simulink model "HUAUV3_"  (R2019a)
settings: Solver=VariableStepAuto  StartTime=0.0  StopTime=30  RelTol=1e-3
InitFcn:
  | run('HUAUVInitial.m')
values from neighbouring files (symbols this model uses):
  buoPos =     [HUAUVPARAMETERS.mat]
  coeff =     [HUAUVPARAMETERS.mat]
  g = 9.8    [HUAUVInitial.m]    (also in HUAUVPARAMETERS.mat)
  Jx = 2.365e-2    (= 0.02365)    [HUAUVInitial.m]    (also in HUAUVPARAMETERS.mat)
  Jy = 1.318e-2    (= 0.01318)    [HUAUVInitial.m]    (also in HUAUVPARAMETERS.mat)
  Jz = 1.318e-2    (= 0.01318)    [HUAUVInitial.m]    (also in HUAUVPARAMETERS.mat)
  m = 1.8    [HUAUVInitial.m]    (also in HUAUVPARAMETERS.mat)
  Sx = 0.07*0.15    (= 0.0105)    [HUAUVInitial.m]    (also in HUAUVPARAMETERS.mat)
  Sy = 0.07*0.28    (= 0.0196)    [HUAUVInitial.m]    (also in HUAUVPARAMETERS.mat)
  Sz = 0.15*0.28    (= 0.042)    [HUAUVInitial.m]    (also in HUAUVPARAMETERS.mat)
  V = 1e-3    (= 0.001)    [HUAUVInitial.m]
undefined symbols (not defined in the file or in its folder): rho
libraries: simulink x12, shared6dof x2
(part 1 of 2)
settings Model: Creator=MI  LastModifiedBy=MI
settings DataIOCC: ReturnWorkspaceOutputs=off
settings DebuggingCC: PregeneratedLibrarySubsystemCodeDiagnostic=none  ArithmeticOperatorsInVariantConditions=warning
settings SFSimCC: SimUseLocalCustomCode=off
settings RTWCC: RTWUseLocalCustomCode=off

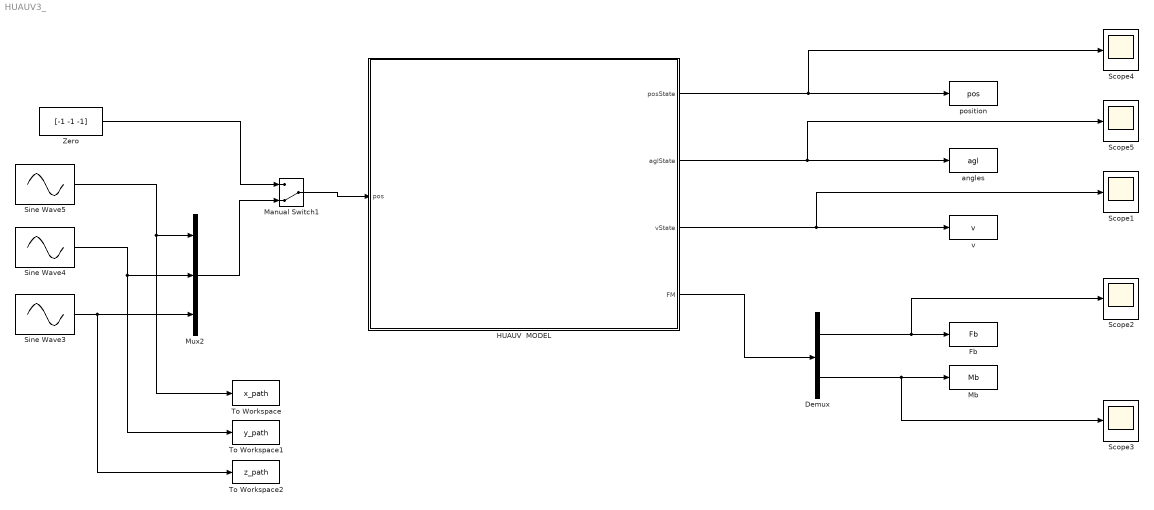
== system HUAUV3_ ==
  Demux : Demux  Outputs=2
  Fb : ToWorkspace  VariableName=Fb  SampleTime=-1
  HUAUV  MODEL : Subsystem
  Manual Switch1 : ManualSwitch  CurrentSetting=0
  Mb : ToWorkspace  VariableName=Mb  SampleTime=-1
  Mux2 : Mux  Inputs=3
  Scope{1..5} (5 alike) : Scope
  Sine Wave3 : Sin  Bias=1  Frequency=0.5  SampleTime=0
  Sine Wave4 : Sin  Frequency=2  Phase=pi/2  SampleTime=0
  Sine Wave5 : Sin  Frequency=2  Phase=pi/3  SampleTime=0
  To Workspace : ToWorkspace  VariableName=x_path  SampleTime=-1
  To Workspace1 : ToWorkspace  VariableName=y_path  SampleTime=-1
  To Workspace2 : ToWorkspace  VariableName=z_path  SampleTime=-1
  Zero : Constant  Value=[-1 -1 -1]
  angles : ToWorkspace  VariableName=agl  SampleTime=-1
  position : ToWorkspace  VariableName=pos  SampleTime=-1
  v : ToWorkspace  VariableName=v  SampleTime=-1
  wires:
  Manual Switch1/1 -> HUAUV  MODEL/1(pos)
  Sine Wave5/1 -> To Workspace/1, Mux2/1
  Sine Wave4/1 -> To Workspace1/1, Mux2/2
  Zero/1 -> Manual Switch1/1
  Mux2/1 -> Manual Switch1/2
  Sine Wave3/1 -> To Workspace2/1, Mux2/3
  HUAUV  MODEL/1(posState) -> position/1, Scope4/1
  HUAUV  MODEL/2(aglState) -> Scope5/1, angles/1
  HUAUV  MODEL/3(vState) -> Scope1/1, v/1
  HUAUV  MODEL/4(FM) -> Demux/1
  Demux/1 -> Scope2/1, Fb/1
  Demux/2 -> Scope3/1, Mb/1

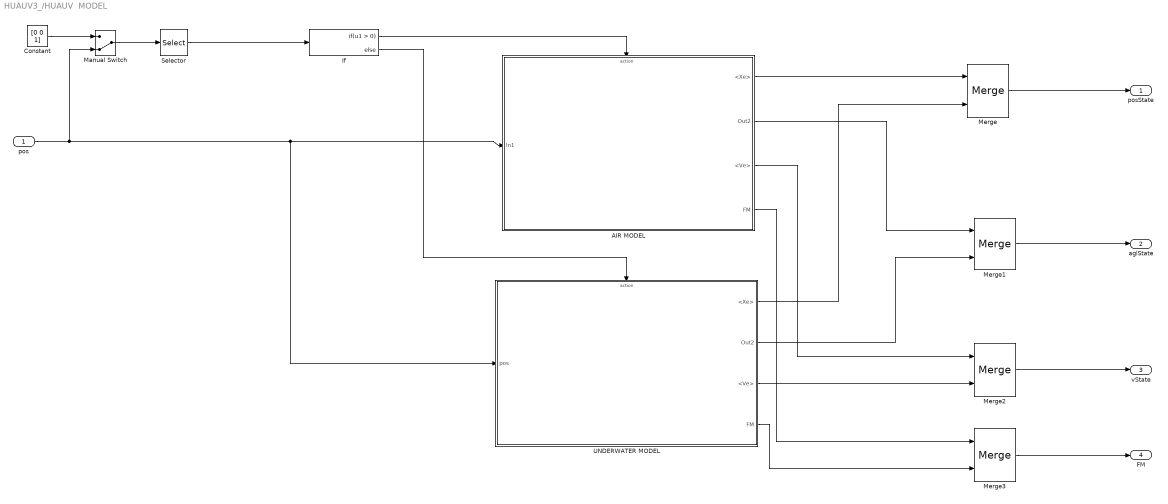
== system HUAUV3_/HUAUV  MODEL ==
  pos : Inport
  AIR MODEL : Subsystem
  Constant : Constant  Value=[0 0 1]
  If : If
  Manual Switch : ManualSwitch  CurrentSetting=0
  Merge{,1..3} (4 alike) : Merge
  Selector : Selector  InputPortWidth=3  IndexOptions=Index vector (dialog)  Indices=[3]  OutputSizes=1
  UNDERWATER MODEL : Subsystem
  posState : Outport
  aglState : Outport  Port=2
  vState : Outport  Port=3
  FM : Outport  Port=4
  wires:
  pos/1 -> Manual Switch/2, UNDERWATER MODEL/1(pos), AIR MODEL/1(In1)
  AIR MODEL/1(<Xe>) -> Merge/1
  UNDERWATER MODEL/1(<Xe>) -> Merge/2
  AIR MODEL/2(Out2) -> Merge1/1
  UNDERWATER MODEL/2(Out2) -> Merge1/2
  Merge1/1 -> aglState/1
  If/1 -> AIR MODEL/Action
  If/2 -> UNDERWATER MODEL/Action
  Manual Switch/1 -> Selector/1
  Merge/1 -> posState/1
  Selector/1 -> If/1
  Constant/1 -> Manual Switch/1
  AIR MODEL/3(<Ve>) -> Merge2/1
  UNDERWATER MODEL/3(<Ve>) -> Merge2/2
  Merge2/1 -> vState/1
  AIR MODEL/4(FM) -> Merge3/1
  UNDERWATER MODEL/4(FM) -> Merge3/2
  Merge3/1 -> FM/1

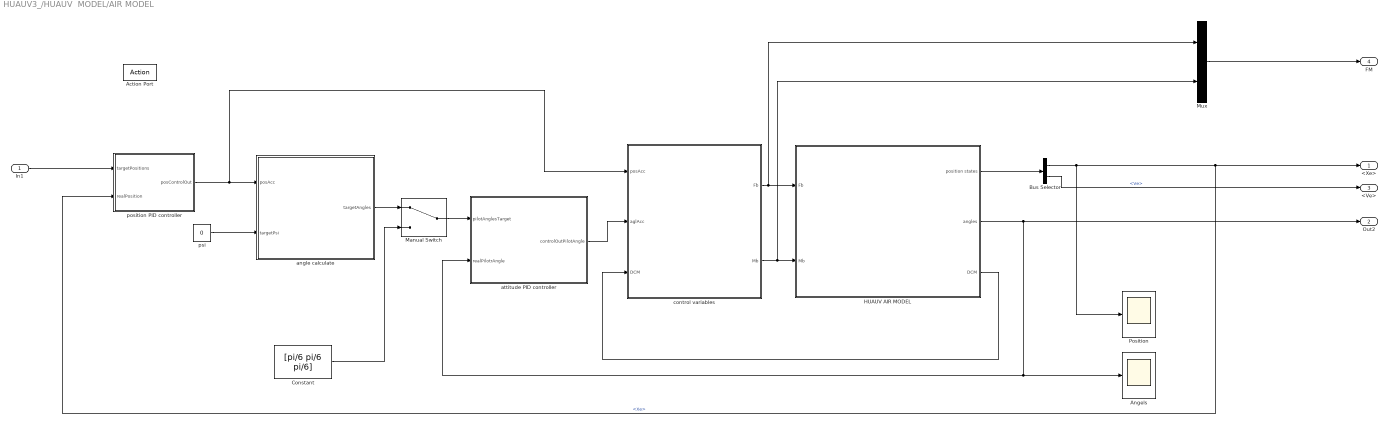
== system HUAUV3_/HUAUV  MODEL/AIR MODEL ==
  In1 : Inport
  Action Port : ActionPort  InitializeStates=reset  ActionPortLabel=if(u1 > 0)
  Angels : Scope
  Bus Selector : BusSelector  OutputSignals=Xe,Ve
  Constant : Constant  Value=[pi/6 pi/6 pi/6]
  HUAUV AIR MODEL : Subsystem
  Manual Switch : ManualSwitch
  Mux : Mux  Inputs=2
  Position : Scope
  angle calculate : Subsystem
  attitude PID controller : Subsystem
  control variables : Subsystem
  position PID controller : Subsystem
  psi : Constant  Value=0
  <Xe> : Outport
  Out2 : Outport  Port=2
  <Ve> : Outport  Port=3
  FM : Outport  Port=4
  wires:
  attitude PID controller/1(controlOutPilotAngle) -> control variables/2(aglAcc)
  position PID controller/1(posControlOut) -> control variables/1(posAcc), angle calculate/1(posAcc)
  psi/1 -> angle calculate/2(targetPsi)
  HUAUV AIR MODEL/1(position states) -> Bus Selector/1
  Constant/1 -> Manual Switch/2
  HUAUV AIR MODEL/3(DCM) -> control variables/3(DCM)
  control variables/2(Mb) -> Mux/2, HUAUV AIR MODEL/2(Mb)
  Manual Switch/1 -> attitude PID controller/1(pilotAnglesTarget)
  HUAUV AIR MODEL/2(angles) -> Out2/1, Angels/1, attitude PID controller/2(realPilotrAngle)
  Bus Selector/1 -> Position/1, position PID controller/2(realPosition), <Xe>/1  "<Xe>"
  angle calculate/1(targetAngles) -> Manual Switch/1
  In1/1 -> position PID controller/1(targetPositions)
  control variables/1(Fb) -> Mux/1, HUAUV AIR MODEL/1(Fb)
  Bus Selector/2 -> <Ve>/1  "<Ve>"
  Mux/1 -> FM/1

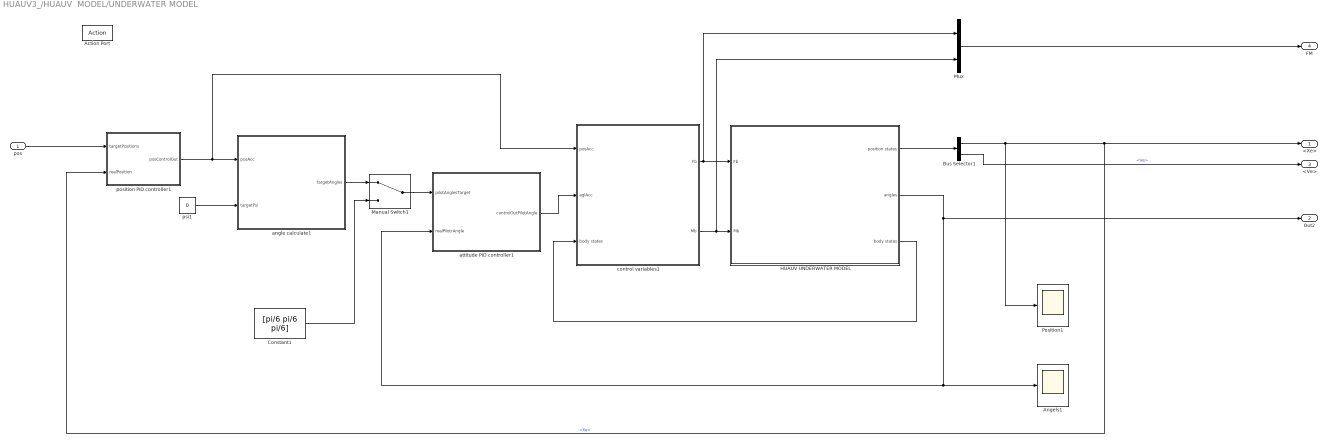
== system HUAUV3_/HUAUV  MODEL/UNDERWATER MODEL ==
  pos : Inport
  Action Port : ActionPort  InitializeStates=reset  ActionPortLabel=else
  Angels1 : Scope
  Bus Selector1 : BusSelector  OutputSignals=Xe,Ve
  Constant1 : Constant  Value=[pi/6 pi/6 pi/6]
  HUAUV UNDERWATER MODEL : Subsystem
  Manual Switch1 : ManualSwitch
  Mux : Mux  Inputs=2
  Position1 : Scope
  angle calculate1 : Subsystem
  attitude PID controller1 : Subsystem
  control variables1 : Subsystem
  position PID controller1 : Subsystem
  psi1 : Constant  Value=0
  <Xe> : Outport
  Out2 : Outport  Port=2
  <Ve> : Outport  Port=3
  FM : Outport  Port=4
  wires:
  position PID controller1/1(posControlOut) -> control variables1/1(posAcc), angle calculate1/1(posAcc)
  HUAUV UNDERWATER MODEL/2(angles) -> Out2/1, Angels1/1, attitude PID controller1/2(realPilotrAngle)
  HUAUV UNDERWATER MODEL/1(position states) -> Bus Selector1/1
  control variables1/1(Fb) -> Mux/1, HUAUV UNDERWATER MODEL/1(Fb)
  psi1/1 -> angle calculate1/2(targetPsi)
  angle calculate1/1(targetAngles) -> Manual Switch1/1
  control variables1/2(Mb) -> Mux/2, HUAUV UNDERWATER MODEL/2(Mb)
  HUAUV UNDERWATER MODEL/3(body states) -> control variables1/3(body states)
  Constant1/1 -> Manual Switch1/2
  attitude PID controller1/1(controlOutPilotAngle) -> control variables1/2(aglAcc)
  Bus Selector1/1 -> Position1/1, position PID controller1/2(realPosition), <Xe>/1  "<Xe>"
  Manual Switch1/1 -> attitude PID controller1/1(pilotAnglesTarget)
  pos/1 -> position PID controller1/1(targetPositions)
  Bus Selector1/2 -> <Ve>/1  "<Ve>"
  Mux/1 -> FM/1

== system HUAUV3_/HUAUV  MODEL/AIR MODEL/HUAUV AIR MODEL ==
  Fb : Inport
  Mb : Inport  Port=2
  Bus Creator : BusCreator  Inputs=3
  HUAUV  6DOF Dynamic Model (Euler Angles) : shared6dof/6DOF (Euler Angles)  units=Metric (MKS)  mtype=Custom Variable  rep=Euler Angles  xme_0=[0 0 0]  Vm_0=[0 0 0]  eul_0=[0 0 0]  pm_0=[0 0 0]  mass_0=1.0  mass_e=0.5  mass_f=2.0  inertia=eye(3)  inertia_e=eye(3)  inertia_f=2*eye(3)  k_quat=1.0  vre_flag=off  abi_flag=on  aMode=0  xme_statename=''  Vm_statename=''  eul_statename=''  quat_statename=''  pm_statename=''  mass_statename=''
      settings: SourceProductBaseCode=AE
  Terminator{1..4} (4 alike) : Terminator
  frame parameters : Subsystem
  position states : Outport
  angles : Outport  Port=2
  DCM : Outport  Port=3
  wires:
  HUAUV  6DOF Dynamic Model (Euler Angles)/2 -> Bus Creator/1  "Xe"
  HUAUV  6DOF Dynamic Model (Euler Angles)/4 -> DCM/1
  HUAUV  6DOF Dynamic Model (Euler Angles)/9 -> Bus Creator/3  "Ae"
  frame parameters/1(m) -> HUAUV  6DOF Dynamic Model (Euler Angles)/3
  HUAUV  6DOF Dynamic Model (Euler Angles)/1 -> Bus Creator/2  "Ve"
  HUAUV  6DOF Dynamic Model (Euler Angles)/7 -> Terminator3/1
  HUAUV  6DOF Dynamic Model (Euler Angles)/5 -> Terminator1/1
  HUAUV  6DOF Dynamic Model (Euler Angles)/8 -> Terminator4/1
  Mb/1 -> HUAUV  6DOF Dynamic Model (Euler Angles)/2
  Bus Creator/1 -> position states/1
  HUAUV  6DOF Dynamic Model (Euler Angles)/6 -> Terminator2/1
  frame parameters/2(dI/dt) -> HUAUV  6DOF Dynamic Model (Euler Angles)/4
  frame parameters/3(I) -> HUAUV  6DOF Dynamic Model (Euler Angles)/5
  Fb/1 -> HUAUV  6DOF Dynamic Model (Euler Angles)/1
  HUAUV  6DOF Dynamic Model (Euler Angles)/3 -> angles/1

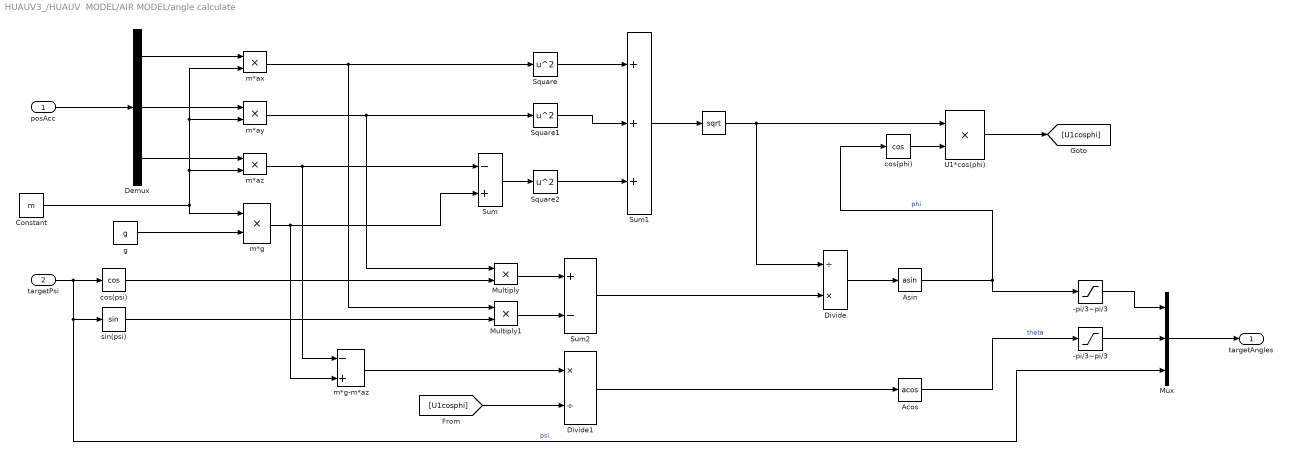
== system HUAUV3_/HUAUV  MODEL/AIR MODEL/angle calculate ==
  posAcc : Inport
  targetPsi : Inport  Port=2
  " " : Sqrt  SaturateOnIntegerOverflow=on
  -pi/3~pi/3 : Saturate  UpperLimit=pi/3  LowerLimit=-pi/3
  "-pi/3~pi/3  " : Saturate  UpperLimit=pi/3  LowerLimit=-pi/3
  Acos : Trigonometry  Operator=acos
  Asin : Trigonometry  Operator=asin
  Constant : Constant  Value=m
  Demux : Demux  Outputs=3
  Divide : Product  Inputs=/*
  Divide1 : Product  Inputs=*/
  Multiply : Product
  Multiply1 : Product
  Mux : Mux  Inputs=3
  Square : Math  Operator=square  SaturateOnIntegerOverflow=on
  Square1 : Math  Operator=square  SaturateOnIntegerOverflow=on
  Square2 : Math  Operator=square  SaturateOnIntegerOverflow=on
  Sum : Sum  Inputs=-+
  Sum1 : Sum  Inputs=+++
  Sum2 : Sum  Inputs=+-
  U1*cos(phi) : Product
  cos(phi) : Trigonometry  Operator=cos
  cos(psi) : Trigonometry  Operator=cos
  g : Constant  Value=g
  m*ax : Product
  m*ay : Product
  m*az : Product
  m*g : Product
  m*g-m*az : Sum  Inputs=-+
  sin(psi) : Trigonometry
  targetAngles : Outport
  wires:
  posAcc/1 -> Demux/1
  Demux/3 -> m*az/1
  Demux/2 -> m*ay/1
  Demux/1 -> m*ax/1
  Constant/1 -> m*g/1, m*ax/2, m*ay/2, m*az/2
  m*ay/1 -> Square1/1, Multiply/1
  m*ax/1 -> Multiply1/1, Square/1
  g/1 -> m*g/2
  m*g/1 -> m*g-m*az/2, Sum/2
  m*az/1 -> m*g-m*az/1, Sum/1
  Sum/1 -> Square2/1
  Square/1 -> Sum1/1
  Square2/1 -> Sum1/3
  Square1/1 -> Sum1/2
  Sum1/1 -> " "/1
  targetPsi/1 -> Mux/3, sin(psi)/1, cos(psi)/1  "psi"
  cos(psi)/1 -> Multiply/2
  sin(psi)/1 -> Multiply1/2
  Multiply1/1 -> Sum2/2
  Multiply/1 -> Sum2/1
  Sum2/1 -> Divide/2
  " "/1 -> Divide/1, U1*cos(phi)/1
  Divide/1 -> Asin/1
  Asin/1 -> -pi/3~pi/3/1, cos(phi)/1  "phi"
  Mux/1 -> targetAngles/1
  Acos/1 -> "-pi/3~pi/3  "/1  "theta"
  cos(phi)/1 -> U1*cos(phi)/2
  U1*cos(phi)/1 -> [U1cosphi]
  m*g-m*az/1 -> Divide1/1
  [U1cosphi] -> Divide1/2
  Divide1/1 -> Acos/1
  -pi/3~pi/3/1 -> Mux/1
  "-pi/3~pi/3  "/1 -> Mux/2

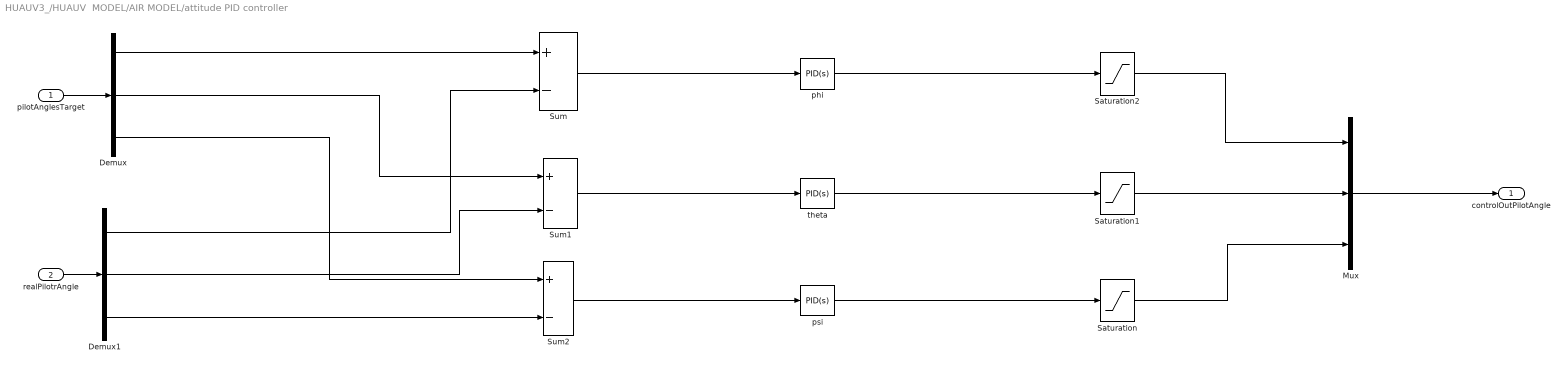
== system HUAUV3_/HUAUV  MODEL/AIR MODEL/attitude PID controller ==
  pilotAnglesTarget : Inport
  realPilotrAngle : Inport  Port=2
  Demux : Demux  Outputs=3
  Demux1 : Demux  Outputs=3
  Mux : Mux  Inputs=3
  Saturation : Saturate  UpperLimit=200  LowerLimit=-200
  Saturation1 : Saturate  UpperLimit=200  LowerLimit=-200
  Saturation2 : Saturate  UpperLimit=200  LowerLimit=-200
  Sum : Sum  Inputs=+-
  Sum1 : Sum  Inputs=+-
  Sum2 : Sum  Inputs=+-
  phi : simulink/Continuous/PID Controller  Controller=PID  Form=Parallel  TimeDomain=Continuous-time  SampleTime=-1  IntegratorMethod=Forward Euler  FilterMethod=Forward Euler  ControllerParametersSource=internal  P=607.007237650316  I=538.5363122748  D=152.017546187089  UseFilter=on  N=17379.6431323802  TunerSelectOption=Transfer Function Based (PID Tuner App)  InitialConditionSource=internal  InitialConditionForIntegrator=0  InitialConditionForFilter=0  DifferentiatorICPrevScaledInput=0  ExternalReset=none  TrackingMode=off  Kt=1  LimitOutput=off  UpperSaturationLimit=inf  LowerSaturationLimit=-inf  LinearizeAsGain=on  AntiWindupMode=none  Kb=1  POutMin=[]  POutMax=[]  IOutMin=[]  IOutMax=[]  DOutMin=[]  DOutMax=[]  NOutMin=[]  NOutMax=[]  SumOutMin=[]  SumOutMax=[]  SaturationOutMin=[]  SaturationOutMax=[]  PParamMin=[]  PParamMax=[]  IParamMin=[]  IParamMax=[]  DParamMin=[]  DParamMax=[]  NParamMin=[]  NParamMax=[]  KbParamMin=[]  KbParamMax=[]  KtParamMin=[]  KtParamMax=[]  KbOutMin=[]  KbOutMax=[]  KtOutMin=[]  KtOutMax=[]  IntegratorOutMin=[]  IntegratorOutMax=[]  FilterOutMin=[]  FilterOutMax=[]  SumI1OutMin=[]  SumI1OutMax=[]  SumI2OutMin=[]  SumI2OutMax=[]  SumI3OutMin=[]  SumI3OutMax=[]  SumI4OutMin=[]  SumI4OutMax=[]  SumDOutMin=[]  SumDOutMax=[]  DifferentiatorOutMin=[]  DifferentiatorOutMax=[]  FilterDiffOutCoefMin=[]  FilterDiffOutCoefMax=[]  ReciprocalOutMin=[]  ReciprocalOutMax=[]  SumDenOutMin=[]  SumDenOutMax=[]  SumNumOutMin=[]  SumNumOutMax=[]  DivideOutMin=[]  DivideOutMax=[]  IntegratorContinuousStateAttributes=''  IntegratorStateMustResolveToSignalObject=off  IntegratorRTWStateStorageClass=Auto  FilterContinuousStateAttributes=''  FilterStateMustResolveToSignalObject=off  FilterRTWStateStorageClass=Auto  ParallelPVariant=InternalParameters  IdealPVariant=Disabled  IVariant=InternalParameters  DVariant=InternalParameters  IntegratorVariant=Continuous  SatVariant=Disabled  AWVariant=Passthrough  PCopyVariant=Disabled  TRVariant=Disabled  FdbkBlocksVariant=Forward  IdealPFdbkVariant=Disabled  SatFdbkVariant=Disabled  DerivativeFilterVariant=ContFilter  NVariant=InternalParameters  NCopyVariant=Disabled  FilterICVariant=InternalICsFilter  IntegratorICVariant=InternalICs  ExternalResetVariant=Disabled  TRSumVariant=Passthrough  SumFdbkVariant=Disabled  SumVariant=Sum_PID
  psi : simulink/Continuous/PID Controller  Controller=PID  Form=Parallel  TimeDomain=Continuous-time  SampleTime=-1  IntegratorMethod=Forward Euler  FilterMethod=Forward Euler  ControllerParametersSource=internal  P=264.968269519038  I=155.315569017994  D=100.436996748118  UseFilter=on  N=11482.6163462738  TunerSelectOption=Transfer Function Based (PID Tuner App)  InitialConditionSource=internal  InitialConditionForIntegrator=0  InitialConditionForFilter=0  DifferentiatorICPrevScaledInput=0  ExternalReset=none  TrackingMode=off  Kt=1  LimitOutput=off  UpperSaturationLimit=inf  LowerSaturationLimit=-inf  LinearizeAsGain=on  AntiWindupMode=none  Kb=1  POutMin=[]  POutMax=[]  IOutMin=[]  IOutMax=[]  DOutMin=[]  DOutMax=[]  NOutMin=[]  NOutMax=[]  SumOutMin=[]  SumOutMax=[]  SaturationOutMin=[]  SaturationOutMax=[]  PParamMin=[]  PParamMax=[]  IParamMin=[]  IParamMax=[]  DParamMin=[]  DParamMax=[]  NParamMin=[]  NParamMax=[]  KbParamMin=[]  KbParamMax=[]  KtParamMin=[]  KtParamMax=[]  KbOutMin=[]  KbOutMax=[]  KtOutMin=[]  KtOutMax=[]  IntegratorOutMin=[]  IntegratorOutMax=[]  FilterOutMin=[]  FilterOutMax=[]  SumI1OutMin=[]  SumI1OutMax=[]  SumI2OutMin=[]  SumI2OutMax=[]  SumI3OutMin=[]  SumI3OutMax=[]  SumI4OutMin=[]  SumI4OutMax=[]  SumDOutMin=[]  SumDOutMax=[]  DifferentiatorOutMin=[]  DifferentiatorOutMax=[]  FilterDiffOutCoefMin=[]  FilterDiffOutCoefMax=[]  ReciprocalOutMin=[]  ReciprocalOutMax=[]  SumDenOutMin=[]  SumDenOutMax=[]  SumNumOutMin=[]  SumNumOutMax=[]  DivideOutMin=[]  DivideOutMax=[]  IntegratorContinuousStateAttributes=''  IntegratorStateMustResolveToSignalObject=off  IntegratorRTWStateStorageClass=Auto  FilterContinuousStateAttributes=''  FilterStateMustResolveToSignalObject=off  FilterRTWStateStorageClass=Auto  ParallelPVariant=InternalParameters  IdealPVariant=Disabled  IVariant=InternalParameters  DVariant=InternalParameters  IntegratorVariant=Continuous  SatVariant=Disabled  AWVariant=Passthrough  PCopyVariant=Disabled  TRVariant=Disabled  FdbkBlocksVariant=Forward  IdealPFdbkVariant=Disabled  SatFdbkVariant=Disabled  DerivativeFilterVariant=ContFilter  NVariant=InternalParameters  NCopyVariant=Disabled  FilterICVariant=InternalICsFilter  IntegratorICVariant=InternalICs  ExternalResetVariant=Disabled  TRSumVariant=Passthrough  SumFdbkVariant=Disabled  SumVariant=Sum_PID
  theta : simulink/Continuous/PID Controller  Controller=PID  Form=Parallel  TimeDomain=Continuous-time  SampleTime=-1  IntegratorMethod=Forward Euler  FilterMethod=Forward Euler  ControllerParametersSource=internal  P=264.968269518041  I=155.31556901741  D=100.43699674774  UseFilter=on  N=11482.6163462738  TunerSelectOption=Transfer Function Based (PID Tuner App)  InitialConditionSource=internal  InitialConditionForIntegrator=0  InitialConditionForFilter=0  DifferentiatorICPrevScaledInput=0  ExternalReset=none  TrackingMode=off  Kt=1  LimitOutput=off  UpperSaturationLimit=inf  LowerSaturationLimit=-inf  LinearizeAsGain=on  AntiWindupMode=none  Kb=1  POutMin=[]  POutMax=[]  IOutMin=[]  IOutMax=[]  DOutMin=[]  DOutMax=[]  NOutMin=[]  NOutMax=[]  SumOutMin=[]  SumOutMax=[]  SaturationOutMin=[]  SaturationOutMax=[]  PParamMin=[]  PParamMax=[]  IParamMin=[]  IParamMax=[]  DParamMin=[]  DParamMax=[]  NParamMin=[]  NParamMax=[]  KbParamMin=[]  KbParamMax=[]  KtParamMin=[]  KtParamMax=[]  KbOutMin=[]  KbOutMax=[]  KtOutMin=[]  KtOutMax=[]  IntegratorOutMin=[]  IntegratorOutMax=[]  FilterOutMin=[]  FilterOutMax=[]  SumI1OutMin=[]  SumI1OutMax=[]  SumI2OutMin=[]  SumI2OutMax=[]  SumI3OutMin=[]  SumI3OutMax=[]  SumI4OutMin=[]  SumI4OutMax=[]  SumDOutMin=[]  SumDOutMax=[]  DifferentiatorOutMin=[]  DifferentiatorOutMax=[]  FilterDiffOutCoefMin=[]  FilterDiffOutCoefMax=[]  ReciprocalOutMin=[]  ReciprocalOutMax=[]  SumDenOutMin=[]  SumDenOutMax=[]  SumNumOutMin=[]  SumNumOutMax=[]  DivideOutMin=[]  DivideOutMax=[]  IntegratorContinuousStateAttributes=''  IntegratorStateMustResolveToSignalObject=off  IntegratorRTWStateStorageClass=Auto  FilterContinuousStateAttributes=''  FilterStateMustResolveToSignalObject=off  FilterRTWStateStorageClass=Auto  ParallelPVariant=InternalParameters  IdealPVariant=Disabled  IVariant=InternalParameters  DVariant=InternalParameters  IntegratorVariant=Continuous  SatVariant=Disabled  AWVariant=Passthrough  PCopyVariant=Disabled  TRVariant=Disabled  FdbkBlocksVariant=Forward  IdealPFdbkVariant=Disabled  SatFdbkVariant=Disabled  DerivativeFilterVariant=ContFilter  NVariant=InternalParameters  NCopyVariant=Disabled  FilterICVariant=InternalICsFilter  IntegratorICVariant=InternalICs  ExternalResetVariant=Disabled  TRSumVariant=Passthrough  SumFdbkVariant=Disabled  SumVariant=Sum_PID
  controlOutPilotAngle : Outport
  wires:
  Sum2/1 -> psi/1
  psi/1 -> Saturation/1
  Demux1/2 -> Sum1/2
  phi/1 -> Saturation2/1
  Demux1/1 -> Sum/2
  Demux/2 -> Sum1/1
  Sum/1 -> phi/1
  Demux/3 -> Sum2/1
  Sum1/1 -> theta/1
  Demux1/3 -> Sum2/2
  theta/1 -> Saturation1/1
  Demux/1 -> Sum/1
  pilotAnglesTarget/1 -> Demux/1
  realPilotrAngle/1 -> Demux1/1
  Mux/1 -> controlOutPilotAngle/1
  Saturation/1 -> Mux/3
  Saturation2/1 -> Mux/1
  Saturation1/1 -> Mux/2

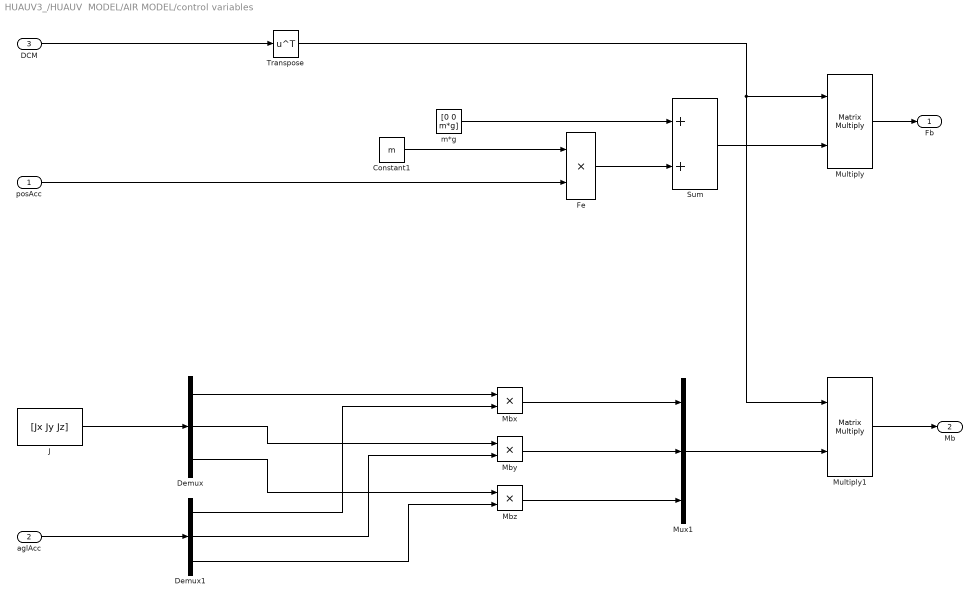
== system HUAUV3_/HUAUV  MODEL/AIR MODEL/control variables ==
  posAcc : Inport
  aglAcc : Inport  Port=2
  DCM : Inport  Port=3
  Constant1 : Constant  Value=m
  Demux : Demux  Outputs=3
  Demux1 : Demux  Outputs=3
  Fe : Product
  J : Constant  Value=[Jx Jy Jz]
  Mbx : Product
  Mby : Product
  Mbz : Product
  Multiply : Product  Multiplication=Matrix(*)
  Multiply1 : Product  Multiplication=Matrix(*)
  Mux1 : Mux  Inputs=3
  Sum : Sum
  Transpose : Math  Operator=transpose  SaturateOnIntegerOverflow=on
  m*g : Constant  Value=[0 0 m*g]
  Fb : Outport
  Mb : Outport  Port=2
  wires:
  Demux/3 -> Mbz/1
  Demux1/2 -> Mby/2
  Demux/2 -> Mby/1
  Demux/1 -> Mbx/1
  Demux1/3 -> Mbz/2
  Demux1/1 -> Mbx/2
  aglAcc/1 -> Demux1/1
  J/1 -> Demux/1
  Mby/1 -> Mux1/2
  Mbx/1 -> Mux1/1
  Mbz/1 -> Mux1/3
  Fe/1 -> Sum/2
  m*g/1 -> Sum/1
  Constant1/1 -> Fe/1
  posAcc/1 -> Fe/2
  Multiply/1 -> Fb/1
  Multiply1/1 -> Mb/1
  Sum/1 -> Multiply/2
  Mux1/1 -> Multiply1/2
  DCM/1 -> Transpose/1
  Transpose/1 -> Multiply1/1, Multiply/1

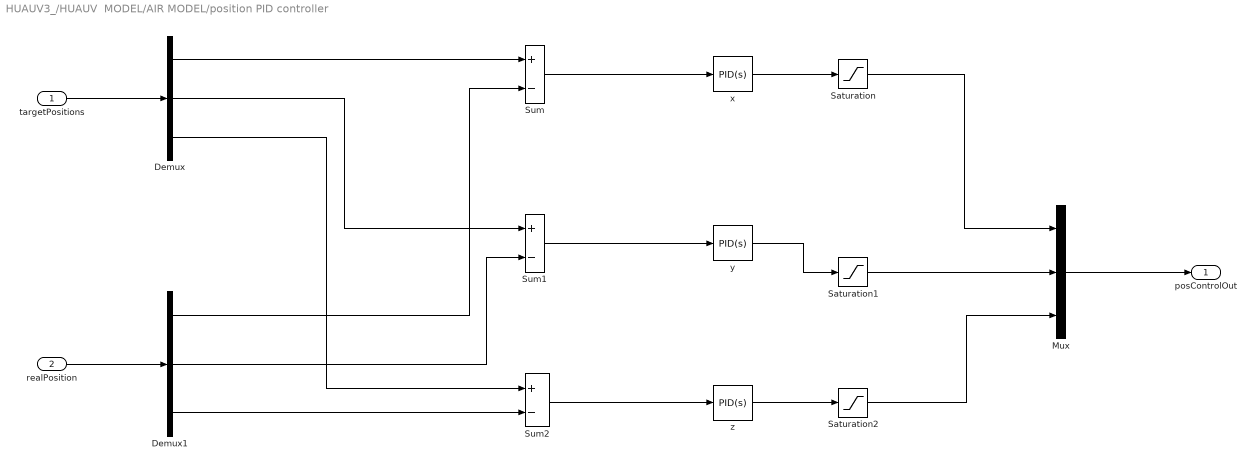
== system HUAUV3_/HUAUV  MODEL/AIR MODEL/position PID controller ==
  targetPositions : Inport
  realPosition : Inport  Port=2
  Demux : Demux  Outputs=3
  Demux1 : Demux  Outputs=3
  Mux : Mux  Inputs=3
  Saturation : Saturate  UpperLimit=100  LowerLimit=-100
  Saturation1 : Saturate  UpperLimit=100  LowerLimit=-100
  Saturation2 : Saturate  UpperLimit=200  LowerLimit=-200
  Sum : Sum  Inputs=+-
  Sum1 : Sum  Inputs=+-
  Sum2 : Sum  Inputs=+-
  x : simulink/Continuous/PID Controller  Controller=PID  Form=Parallel  TimeDomain=Continuous-time  SampleTime=-1  IntegratorMethod=Forward Euler  FilterMethod=Forward Euler  ControllerParametersSource=internal  P=166.392550246094  I=77.2903021557012  D=79.5909562085375  UseFilter=on  N=9099.36023942606  TunerSelectOption=Transfer Function Based (PID Tuner App)  InitialConditionSource=internal  InitialConditionForIntegrator=0  InitialConditionForFilter=0  DifferentiatorICPrevScaledInput=0  ExternalReset=none  TrackingMode=off  Kt=1  LimitOutput=off  UpperSaturationLimit=inf  LowerSaturationLimit=-inf  LinearizeAsGain=on  AntiWindupMode=none  Kb=1  POutMin=[]  POutMax=[]  IOutMin=[]  IOutMax=[]  DOutMin=[]  DOutMax=[]  NOutMin=[]  NOutMax=[]  SumOutMin=[]  SumOutMax=[]  SaturationOutMin=[]  SaturationOutMax=[]  PParamMin=[]  PParamMax=[]  IParamMin=[]  IParamMax=[]  DParamMin=[]  DParamMax=[]  NParamMin=[]  NParamMax=[]  KbParamMin=[]  KbParamMax=[]  KtParamMin=[]  KtParamMax=[]  KbOutMin=[]  KbOutMax=[]  KtOutMin=[]  KtOutMax=[]  IntegratorOutMin=[]  IntegratorOutMax=[]  FilterOutMin=[]  FilterOutMax=[]  SumI1OutMin=[]  SumI1OutMax=[]  SumI2OutMin=[]  SumI2OutMax=[]  SumI3OutMin=[]  SumI3OutMax=[]  SumI4OutMin=[]  SumI4OutMax=[]  SumDOutMin=[]  SumDOutMax=[]  DifferentiatorOutMin=[]  DifferentiatorOutMax=[]  FilterDiffOutCoefMin=[]  FilterDiffOutCoefMax=[]  ReciprocalOutMin=[]  ReciprocalOutMax=[]  SumDenOutMin=[]  SumDenOutMax=[]  SumNumOutMin=[]  SumNumOutMax=[]  DivideOutMin=[]  DivideOutMax=[]  IntegratorContinuousStateAttributes=''  IntegratorStateMustResolveToSignalObject=off  IntegratorRTWStateStorageClass=Auto  FilterContinuousStateAttributes=''  FilterStateMustResolveToSignalObject=off  FilterRTWStateStorageClass=Auto  ParallelPVariant=InternalParameters  IdealPVariant=Disabled  IVariant=InternalParameters  DVariant=InternalParameters  IntegratorVariant=Continuous  SatVariant=Disabled  AWVariant=Passthrough  PCopyVariant=Disabled  TRVariant=Disabled  FdbkBlocksVariant=Forward  IdealPFdbkVariant=Disabled  SatFdbkVariant=Disabled  DerivativeFilterVariant=ContFilter  NVariant=InternalParameters  NCopyVariant=Disabled  FilterICVariant=InternalICsFilter  IntegratorICVariant=InternalICs  ExternalResetVariant=Disabled  TRSumVariant=Passthrough  SumFdbkVariant=Disabled  SumVariant=Sum_PID
  y : simulink/Continuous/PID Controller  Controller=PID  Form=Parallel  TimeDomain=Continuous-time  SampleTime=-1  IntegratorMethod=Forward Euler  FilterMethod=Forward Euler  ControllerParametersSource=internal  P=263.714420161278  I=154.214427203828  D=100.199077319925  UseFilter=on  N=11455.4158364829  TunerSelectOption=Transfer Function Based (PID Tuner App)  InitialConditionSource=internal  InitialConditionForIntegrator=0  InitialConditionForFilter=0  DifferentiatorICPrevScaledInput=0  ExternalReset=none  TrackingMode=off  Kt=1  LimitOutput=off  UpperSaturationLimit=inf  LowerSaturationLimit=-inf  LinearizeAsGain=on  AntiWindupMode=none  Kb=1  POutMin=[]  POutMax=[]  IOutMin=[]  IOutMax=[]  DOutMin=[]  DOutMax=[]  NOutMin=[]  NOutMax=[]  SumOutMin=[]  SumOutMax=[]  SaturationOutMin=[]  SaturationOutMax=[]  PParamMin=[]  PParamMax=[]  IParamMin=[]  IParamMax=[]  DParamMin=[]  DParamMax=[]  NParamMin=[]  NParamMax=[]  KbParamMin=[]  KbParamMax=[]  KtParamMin=[]  KtParamMax=[]  KbOutMin=[]  KbOutMax=[]  KtOutMin=[]  KtOutMax=[]  IntegratorOutMin=[]  IntegratorOutMax=[]  FilterOutMin=[]  FilterOutMax=[]  SumI1OutMin=[]  SumI1OutMax=[]  SumI2OutMin=[]  SumI2OutMax=[]  SumI3OutMin=[]  SumI3OutMax=[]  SumI4OutMin=[]  SumI4OutMax=[]  SumDOutMin=[]  SumDOutMax=[]  DifferentiatorOutMin=[]  DifferentiatorOutMax=[]  FilterDiffOutCoefMin=[]  FilterDiffOutCoefMax=[]  ReciprocalOutMin=[]  ReciprocalOutMax=[]  SumDenOutMin=[]  SumDenOutMax=[]  SumNumOutMin=[]  SumNumOutMax=[]  DivideOutMin=[]  DivideOutMax=[]  IntegratorContinuousStateAttributes=''  IntegratorStateMustResolveToSignalObject=off  IntegratorRTWStateStorageClass=Auto  FilterContinuousStateAttributes=''  FilterStateMustResolveToSignalObject=off  FilterRTWStateStorageClass=Auto  ParallelPVariant=InternalParameters  IdealPVariant=Disabled  IVariant=InternalParameters  DVariant=InternalParameters  IntegratorVariant=Continuous  SatVariant=Disabled  AWVariant=Passthrough  PCopyVariant=Disabled  TRVariant=Disabled  FdbkBlocksVariant=Forward  IdealPFdbkVariant=Disabled  SatFdbkVariant=Disabled  DerivativeFilterVariant=ContFilter  NVariant=InternalParameters  NCopyVariant=Disabled  FilterICVariant=InternalICsFilter  IntegratorICVariant=InternalICs  ExternalResetVariant=Disabled  TRSumVariant=Passthrough  SumFdbkVariant=Disabled  SumVariant=Sum_PID
  z : simulink/Continuous/PID Controller  Controller=PID  Form=Parallel  TimeDomain=Continuous-time  SampleTime=-1  IntegratorMethod=Forward Euler  FilterMethod=Forward Euler  ControllerParametersSource=internal  P=317.054468255658  I=203.294207844063  D=109.866103554962  UseFilter=on  N=12560.6136924569  TunerSelectOption=Transfer Function Based (PID Tuner App)  InitialConditionSource=internal  InitialConditionForIntegrator=0  InitialConditionForFilter=0  DifferentiatorICPrevScaledInput=0  ExternalReset=none  TrackingMode=off  Kt=1  LimitOutput=off  UpperSaturationLimit=inf  LowerSaturationLimit=-inf  LinearizeAsGain=on  AntiWindupMode=none  Kb=1  POutMin=[]  POutMax=[]  IOutMin=[]  IOutMax=[]  DOutMin=[]  DOutMax=[]  NOutMin=[]  NOutMax=[]  SumOutMin=[]  SumOutMax=[]  SaturationOutMin=[]  SaturationOutMax=[]  PParamMin=[]  PParamMax=[]  IParamMin=[]  IParamMax=[]  DParamMin=[]  DParamMax=[]  NParamMin=[]  NParamMax=[]  KbParamMin=[]  KbParamMax=[]  KtParamMin=[]  KtParamMax=[]  KbOutMin=[]  KbOutMax=[]  KtOutMin=[]  KtOutMax=[]  IntegratorOutMin=[]  IntegratorOutMax=[]  FilterOutMin=[]  FilterOutMax=[]  SumI1OutMin=[]  SumI1OutMax=[]  SumI2OutMin=[]  SumI2OutMax=[]  SumI3OutMin=[]  SumI3OutMax=[]  SumI4OutMin=[]  SumI4OutMax=[]  SumDOutMin=[]  SumDOutMax=[]  DifferentiatorOutMin=[]  DifferentiatorOutMax=[]  FilterDiffOutCoefMin=[]  FilterDiffOutCoefMax=[]  ReciprocalOutMin=[]  ReciprocalOutMax=[]  SumDenOutMin=[]  SumDenOutMax=[]  SumNumOutMin=[]  SumNumOutMax=[]  DivideOutMin=[]  DivideOutMax=[]  IntegratorContinuousStateAttributes=''  IntegratorStateMustResolveToSignalObject=off  IntegratorRTWStateStorageClass=Auto  FilterContinuousStateAttributes=''  FilterStateMustResolveToSignalObject=off  FilterRTWStateStorageClass=Auto  ParallelPVariant=InternalParameters  IdealPVariant=Disabled  IVariant=InternalParameters  DVariant=InternalParameters  IntegratorVariant=Continuous  SatVariant=Disabled  AWVariant=Passthrough  PCopyVariant=Disabled  TRVariant=Disabled  FdbkBlocksVariant=Forward  IdealPFdbkVariant=Disabled  SatFdbkVariant=Disabled  DerivativeFilterVariant=ContFilter  NVariant=InternalParameters  NCopyVariant=Disabled  FilterICVariant=InternalICsFilter  IntegratorICVariant=InternalICs  ExternalResetVariant=Disabled  TRSumVariant=Passthrough  SumFdbkVariant=Disabled  SumVariant=Sum_PID
  posControlOut : Outport
  wires:
  Sum1/1 -> y/1
  y/1 -> Saturation1/1
  Demux1/2 -> Sum1/2
  Demux/3 -> Sum2/1
  Demux/2 -> Sum1/1
  Demux/1 -> Sum/1
  Sum/1 -> x/1
  z/1 -> Saturation2/1
  Sum2/1 -> z/1
  Demux1/3 -> Sum2/2
  targetPositions/1 -> Demux/1
  realPosition/1 -> Demux1/1
  Mux/1 -> posControlOut/1
  x/1 -> Saturation/1
  Saturation/1 -> Mux/1
  Saturation1/1 -> Mux/2
  Saturation2/1 -> Mux/3
  Demux1/1 -> Sum/2

== system HUAUV3_/HUAUV  MODEL/UNDERWATER MODEL/HUAUV UNDERWATER MODEL ==
  Fb : Inport
  Mb : Inport  Port=2
  Bus Creator : BusCreator  Inputs=3
  Bus Creator1 : BusCreator  Inputs=4
  HUAUV  6DOF Dynamic Model (Euler Angles) : shared6dof/6DOF (Euler Angles)  units=Metric (MKS)  mtype=Custom Variable  rep=Euler Angles  xme_0=[0 0 0]  Vm_0=[0 0 0]  eul_0=[0 0 0]  pm_0=[0 0 0]  mass_0=1.0  mass_e=0.5  mass_f=2.0  inertia=eye(3)  inertia_e=eye(3)  inertia_f=2*eye(3)  k_quat=1.0  vre_flag=off  abi_flag=on  aMode=0  xme_statename=''  Vm_statename=''  eul_statename=''  quat_statename=''  pm_statename=''  mass_statename=''
      settings: SourceProductBaseCode=AE
  Terminator3 : Terminator
  Terminator4 : Terminator
  frame parameters : Subsystem
  position states : Outport
  angles : Outport  Port=2
  body states : Outport  Port=3
  wires:
  HUAUV  6DOF Dynamic Model (Euler Angles)/2 -> Bus Creator/1  "Xe"
  HUAUV  6DOF Dynamic Model (Euler Angles)/9 -> Bus Creator/3  "Ae"
  frame parameters/1(m) -> HUAUV  6DOF Dynamic Model (Euler Angles)/3
  HUAUV  6DOF Dynamic Model (Euler Angles)/1 -> Bus Creator/2  "Ve"
  HUAUV  6DOF Dynamic Model (Euler Angles)/7 -> Terminator3/1
  HUAUV  6DOF Dynamic Model (Euler Angles)/8 -> Terminator4/1
  Mb/1 -> HUAUV  6DOF Dynamic Model (Euler Angles)/2
  Bus Creator/1 -> position states/1
  frame parameters/2(dI/dt) -> HUAUV  6DOF Dynamic Model (Euler Angles)/4
  frame parameters/3(I) -> HUAUV  6DOF Dynamic Model (Euler Angles)/5
  Fb/1 -> HUAUV  6DOF Dynamic Model (Euler Angles)/1
  HUAUV  6DOF Dynamic Model (Euler Angles)/3 -> angles/1, Bus Creator1/1  "angle"
  Bus Creator1/1 -> body states/1
  HUAUV  6DOF Dynamic Model (Euler Angles)/6 -> Bus Creator1/4  "Wb"
  HUAUV  6DOF Dynamic Model (Euler Angles)/5 -> Bus Creator1/3  "Vb"
  HUAUV  6DOF Dynamic Model (Euler Angles)/4 -> Bus Creator1/2  "DCMbe"

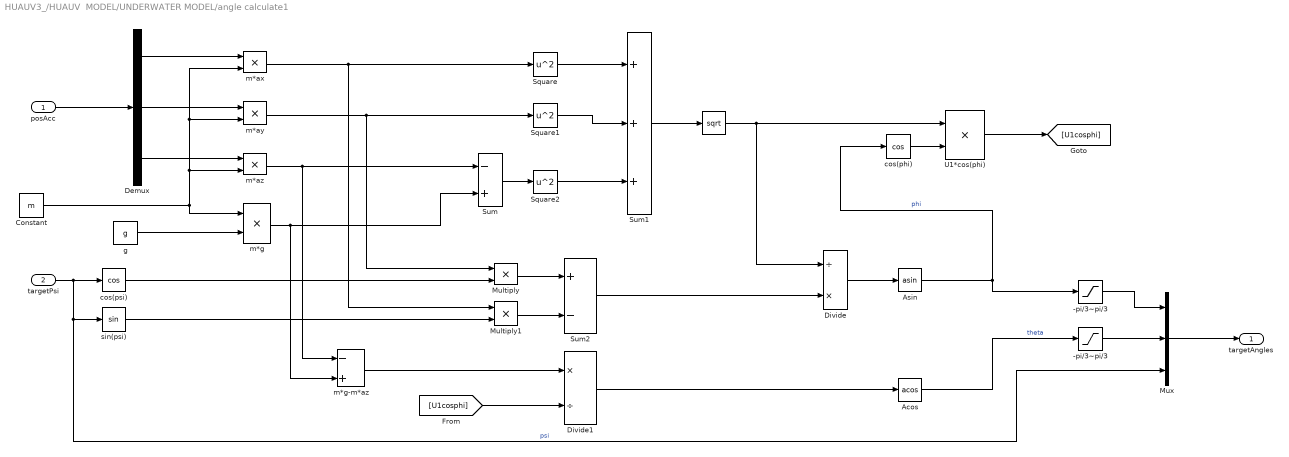
== system HUAUV3_/HUAUV  MODEL/UNDERWATER MODEL/angle calculate1 ==
  posAcc : Inport
  targetPsi : Inport  Port=2
  " " : Sqrt  SaturateOnIntegerOverflow=on
  -pi/3~pi/3 : Saturate  UpperLimit=pi/3  LowerLimit=-pi/3
  "-pi/3~pi/3  " : Saturate  UpperLimit=pi/3  LowerLimit=-pi/3
  Acos : Trigonometry  Operator=acos
  Asin : Trigonometry  Operator=asin
  Constant : Constant  Value=m
  Demux : Demux  Outputs=3
  Divide : Product  Inputs=/*
  Divide1 : Product  Inputs=*/
  Multiply : Product
  Multiply1 : Product
  Mux : Mux  Inputs=3
  Square : Math  Operator=square  SaturateOnIntegerOverflow=on
  Square1 : Math  Operator=square  SaturateOnIntegerOverflow=on
  Square2 : Math  Operator=square  SaturateOnIntegerOverflow=on
  Sum : Sum  Inputs=-+
  Sum1 : Sum  Inputs=+++
  Sum2 : Sum  Inputs=+-
  U1*cos(phi) : Product
  cos(phi) : Trigonometry  Operator=cos
  cos(psi) : Trigonometry  Operator=cos
  g : Constant  Value=g
  m*ax : Product
  m*ay : Product
  m*az : Product
  m*g : Product
  m*g-m*az : Sum  Inputs=-+
  sin(psi) : Trigonometry
  targetAngles : Outport
  wires:
  posAcc/1 -> Demux/1
  Demux/3 -> m*az/1
  Demux/2 -> m*ay/1
  Demux/1 -> m*ax/1
  Constant/1 -> m*g/1, m*ax/2, m*ay/2, m*az/2
  m*ay/1 -> Square1/1, Multiply/1
  m*ax/1 -> Multiply1/1, Square/1
  g/1 -> m*g/2
  m*g/1 -> m*g-m*az/2, Sum/2
  m*az/1 -> m*g-m*az/1, Sum/1
  Sum/1 -> Square2/1
  Square/1 -> Sum1/1
  Square2/1 -> Sum1/3
  Square1/1 -> Sum1/2
  Sum1/1 -> " "/1
  targetPsi/1 -> Mux/3, sin(psi)/1, cos(psi)/1  "psi"
  cos(psi)/1 -> Multiply/2
  sin(psi)/1 -> Multiply1/2
  Multiply1/1 -> Sum2/2
  Multiply/1 -> Sum2/1
  Sum2/1 -> Divide/2
  " "/1 -> Divide/1, U1*cos(phi)/1
  Divide/1 -> Asin/1
  Asin/1 -> -pi/3~pi/3/1, cos(phi)/1  "phi"
  Mux/1 -> targetAngles/1
  Acos/1 -> "-pi/3~pi/3  "/1  "theta"
  cos(phi)/1 -> U1*cos(phi)/2
  U1*cos(phi)/1 -> [U1cosphi]
  m*g-m*az/1 -> Divide1/1
  [U1cosphi] -> Divide1/2
  Divide1/1 -> Acos/1
  -pi/3~pi/3/1 -> Mux/1
  "-pi/3~pi/3  "/1 -> Mux/2

== system HUAUV3_/HUAUV  MODEL/UNDERWATER MODEL/attitude PID controller1 ==
  pilotAnglesTarget : Inport
  realPilotrAngle : Inport  Port=2
  Demux : Demux  Outputs=3
  Demux1 : Demux  Outputs=3
  Mux : Mux  Inputs=3
  Saturation : Saturate  UpperLimit=80  LowerLimit=-80
  Saturation1 : Saturate  UpperLimit=100  LowerLimit=-100
  Saturation2 : Saturate  UpperLimit=100  LowerLimit=-100
  Sum : Sum  Inputs=+-
  Sum1 : Sum  Inputs=+-
  Sum2 : Sum  Inputs=+-
  phi : simulink/Continuous/PID Controller  Controller=PID  Form=Parallel  TimeDomain=Continuous-time  SampleTime=-1  IntegratorMethod=Forward Euler  FilterMethod=Forward Euler  ControllerParametersSource=internal  P=607.007237650316  I=538.5363122748  D=152.017546187089  UseFilter=on  N=17379.6431323802  TunerSelectOption=Transfer Function Based (PID Tuner App)  InitialConditionSource=internal  InitialConditionForIntegrator=0  InitialConditionForFilter=0  DifferentiatorICPrevScaledInput=0  ExternalReset=none  TrackingMode=off  Kt=1  LimitOutput=off  UpperSaturationLimit=inf  LowerSaturationLimit=-inf  LinearizeAsGain=on  AntiWindupMode=none  Kb=1  POutMin=[]  POutMax=[]  IOutMin=[]  IOutMax=[]  DOutMin=[]  DOutMax=[]  NOutMin=[]  NOutMax=[]  SumOutMin=[]  SumOutMax=[]  SaturationOutMin=[]  SaturationOutMax=[]  PParamMin=[]  PParamMax=[]  IParamMin=[]  IParamMax=[]  DParamMin=[]  DParamMax=[]  NParamMin=[]  NParamMax=[]  KbParamMin=[]  KbParamMax=[]  KtParamMin=[]  KtParamMax=[]  KbOutMin=[]  KbOutMax=[]  KtOutMin=[]  KtOutMax=[]  IntegratorOutMin=[]  IntegratorOutMax=[]  FilterOutMin=[]  FilterOutMax=[]  SumI1OutMin=[]  SumI1OutMax=[]  SumI2OutMin=[]  SumI2OutMax=[]  SumI3OutMin=[]  SumI3OutMax=[]  SumI4OutMin=[]  SumI4OutMax=[]  SumDOutMin=[]  SumDOutMax=[]  DifferentiatorOutMin=[]  DifferentiatorOutMax=[]  FilterDiffOutCoefMin=[]  FilterDiffOutCoefMax=[]  ReciprocalOutMin=[]  ReciprocalOutMax=[]  SumDenOutMin=[]  SumDenOutMax=[]  SumNumOutMin=[]  SumNumOutMax=[]  DivideOutMin=[]  DivideOutMax=[]  IntegratorContinuousStateAttributes=''  IntegratorStateMustResolveToSignalObject=off  IntegratorRTWStateStorageClass=Auto  FilterContinuousStateAttributes=''  FilterStateMustResolveToSignalObject=off  FilterRTWStateStorageClass=Auto  ParallelPVariant=InternalParameters  IdealPVariant=Disabled  IVariant=InternalParameters  DVariant=InternalParameters  IntegratorVariant=Continuous  SatVariant=Disabled  AWVariant=Passthrough  PCopyVariant=Disabled  TRVariant=Disabled  FdbkBlocksVariant=Forward  IdealPFdbkVariant=Disabled  SatFdbkVariant=Disabled  DerivativeFilterVariant=ContFilter  NVariant=InternalParameters  NCopyVariant=Disabled  FilterICVariant=InternalICsFilter  IntegratorICVariant=InternalICs  ExternalResetVariant=Disabled  TRSumVariant=Passthrough  SumFdbkVariant=Disabled  SumVariant=Sum_PID
  psi : simulink/Continuous/PID Controller  Controller=PID  Form=Parallel  TimeDomain=Continuous-time  SampleTime=-1  IntegratorMethod=Forward Euler  FilterMethod=Forward Euler  ControllerParametersSource=internal  P=264.968269519038  I=155.315569017994  D=100.436996748118  UseFilter=on  N=11482.6163462738  TunerSelectOption=Transfer Function Based (PID Tuner App)  InitialConditionSource=internal  InitialConditionForIntegrator=0  InitialConditionForFilter=0  DifferentiatorICPrevScaledInput=0  ExternalReset=none  TrackingMode=off  Kt=1  LimitOutput=off  UpperSaturationLimit=inf  LowerSaturationLimit=-inf  LinearizeAsGain=on  AntiWindupMode=none  Kb=1  POutMin=[]  POutMax=[]  IOutMin=[]  IOutMax=[]  DOutMin=[]  DOutMax=[]  NOutMin=[]  NOutMax=[]  SumOutMin=[]  SumOutMax=[]  SaturationOutMin=[]  SaturationOutMax=[]  PParamMin=[]  PParamMax=[]  IParamMin=[]  IParamMax=[]  DParamMin=[]  DParamMax=[]  NParamMin=[]  NParamMax=[]  KbParamMin=[]  KbParamMax=[]  KtParamMin=[]  KtParamMax=[]  KbOutMin=[]  KbOutMax=[]  KtOutMin=[]  KtOutMax=[]  IntegratorOutMin=[]  IntegratorOutMax=[]  FilterOutMin=[]  FilterOutMax=[]  SumI1OutMin=[]  SumI1OutMax=[]  SumI2OutMin=[]  SumI2OutMax=[]  SumI3OutMin=[]  SumI3OutMax=[]  SumI4OutMin=[]  SumI4OutMax=[]  SumDOutMin=[]  SumDOutMax=[]  DifferentiatorOutMin=[]  DifferentiatorOutMax=[]  FilterDiffOutCoefMin=[]  FilterDiffOutCoefMax=[]  ReciprocalOutMin=[]  ReciprocalOutMax=[]  SumDenOutMin=[]  SumDenOutMax=[]  SumNumOutMin=[]  SumNumOutMax=[]  DivideOutMin=[]  DivideOutMax=[]  IntegratorContinuousStateAttributes=''  IntegratorStateMustResolveToSignalObject=off  IntegratorRTWStateStorageClass=Auto  FilterContinuousStateAttributes=''  FilterStateMustResolveToSignalObject=off  FilterRTWStateStorageClass=Auto  ParallelPVariant=InternalParameters  IdealPVariant=Disabled  IVariant=InternalParameters  DVariant=InternalParameters  IntegratorVariant=Continuous  SatVariant=Disabled  AWVariant=Passthrough  PCopyVariant=Disabled  TRVariant=Disabled  FdbkBlocksVariant=Forward  IdealPFdbkVariant=Disabled  SatFdbkVariant=Disabled  DerivativeFilterVariant=ContFilter  NVariant=InternalParameters  NCopyVariant=Disabled  FilterICVariant=InternalICsFilter  IntegratorICVariant=InternalICs  ExternalResetVariant=Disabled  TRSumVariant=Passthrough  SumFdbkVariant=Disabled  SumVariant=Sum_PID
  theta : simulink/Continuous/PID Controller  Controller=PID  Form=Parallel  TimeDomain=Continuous-time  SampleTime=-1  IntegratorMethod=Forward Euler  FilterMethod=Forward Euler  ControllerParametersSource=internal  P=264.968269518041  I=155.31556901741  D=100.43699674774  UseFilter=on  N=11482.6163462738  TunerSelectOption=Transfer Function Based (PID Tuner App)  InitialConditionSource=internal  InitialConditionForIntegrator=0  InitialConditionForFilter=0  DifferentiatorICPrevScaledInput=0  ExternalReset=none  TrackingMode=off  Kt=1  LimitOutput=off  UpperSaturationLimit=inf  LowerSaturationLimit=-inf  LinearizeAsGain=on  AntiWindupMode=none  Kb=1  POutMin=[]  POutMax=[]  IOutMin=[]  IOutMax=[]  DOutMin=[]  DOutMax=[]  NOutMin=[]  NOutMax=[]  SumOutMin=[]  SumOutMax=[]  SaturationOutMin=[]  SaturationOutMax=[]  PParamMin=[]  PParamMax=[]  IParamMin=[]  IParamMax=[]  DParamMin=[]  DParamMax=[]  NParamMin=[]  NParamMax=[]  KbParamMin=[]  KbParamMax=[]  KtParamMin=[]  KtParamMax=[]  KbOutMin=[]  KbOutMax=[]  KtOutMin=[]  KtOutMax=[]  IntegratorOutMin=[]  IntegratorOutMax=[]  FilterOutMin=[]  FilterOutMax=[]  SumI1OutMin=[]  SumI1OutMax=[]  SumI2OutMin=[]  SumI2OutMax=[]  SumI3OutMin=[]  SumI3OutMax=[]  SumI4OutMin=[]  SumI4OutMax=[]  SumDOutMin=[]  SumDOutMax=[]  DifferentiatorOutMin=[]  DifferentiatorOutMax=[]  FilterDiffOutCoefMin=[]  FilterDiffOutCoefMax=[]  ReciprocalOutMin=[]  ReciprocalOutMax=[]  SumDenOutMin=[]  SumDenOutMax=[]  SumNumOutMin=[]  SumNumOutMax=[]  DivideOutMin=[]  DivideOutMax=[]  IntegratorContinuousStateAttributes=''  IntegratorStateMustResolveToSignalObject=off  IntegratorRTWStateStorageClass=Auto  FilterContinuousStateAttributes=''  FilterStateMustResolveToSignalObject=off  FilterRTWStateStorageClass=Auto  ParallelPVariant=InternalParameters  IdealPVariant=Disabled  IVariant=InternalParameters  DVariant=InternalParameters  IntegratorVariant=Continuous  SatVariant=Disabled  AWVariant=Passthrough  PCopyVariant=Disabled  TRVariant=Disabled  FdbkBlocksVariant=Forward  IdealPFdbkVariant=Disabled  SatFdbkVariant=Disabled  DerivativeFilterVariant=ContFilter  NVariant=InternalParameters  NCopyVariant=Disabled  FilterICVariant=InternalICsFilter  IntegratorICVariant=InternalICs  ExternalResetVariant=Disabled  TRSumVariant=Passthrough  SumFdbkVariant=Disabled  SumVariant=Sum_PID
  controlOutPilotAngle : Outport
  wires:
  Sum2/1 -> psi/1
  psi/1 -> Saturation/1
  Demux1/2 -> Sum1/2
  phi/1 -> Saturation2/1
  Demux1/1 -> Sum/2
  Demux/2 -> Sum1/1
  Sum/1 -> phi/1
  Demux/3 -> Sum2/1
  Sum1/1 -> theta/1
  Demux1/3 -> Sum2/2
  theta/1 -> Saturation1/1
  Demux/1 -> Sum/1
  pilotAnglesTarget/1 -> Demux/1
  realPilotrAngle/1 -> Demux1/1
  Mux/1 -> controlOutPilotAngle/1
  Saturation/1 -> Mux/3
  Saturation2/1 -> Mux/1
  Saturation1/1 -> Mux/2

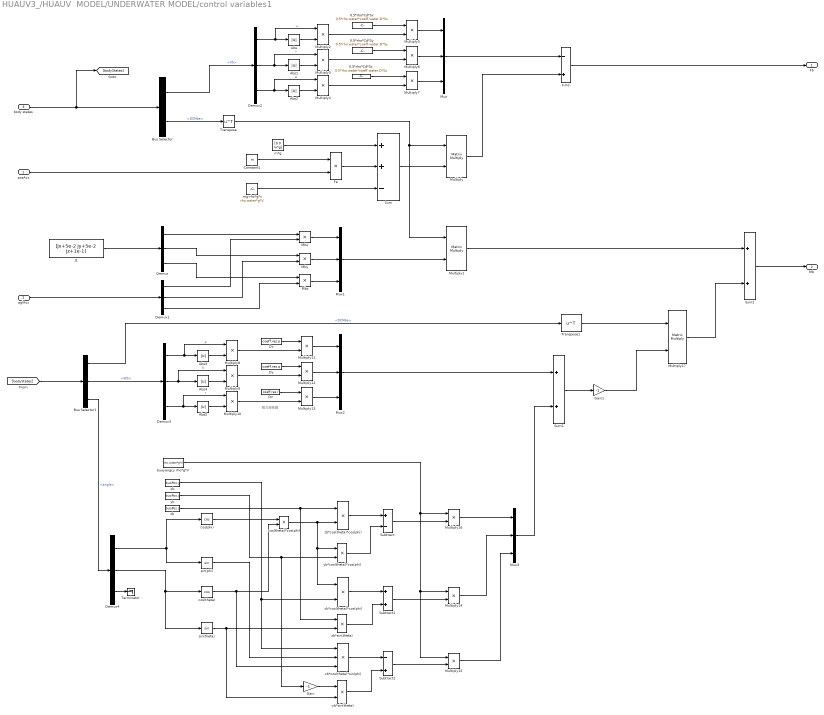
== system HUAUV3_/HUAUV  MODEL/UNDERWATER MODEL/control variables1 ==
  note: 阻力矩系数
  posAcc : Inport
  aglAcc : Inport  Port=2
  body states : Inport  Port=3
  -yb*sin(theta) : Product
  0.5*rho*Cd*Sx : Constant  Value=0.5*rho.water*coeff.water.D*Sx
  0.5*rho*Cd*Sy : Constant  Value=0.5*rho.water*coeff.water.D*Sy
  0.5*rho*Cd*Sz : Constant  Value=0.5*rho.water*coeff.water.D*Sz
  Abs{,1..5} (6 alike) : Abs
  Bus Selector : BusSelector  OutputSignals=Vb,DCMbe
  Bus Selector1 : BusSelector  OutputSignals=DCMbe,Wb,angle
  Constant1 : Constant  Value=m
  Demux{,1..4} (5 alike) : Demux  Outputs=3
  Dx : Constant  Value=coeff.res.p
  Dy : Constant  Value=coeff.res.q
  Dz : Constant  Value=coeff.res.r
  F-Fd : Sum  Inputs=-+
  Fe : Product
  Gain : Gain  Gain=-1
  Gain1 : Gain  Gain=-1
  J1 : Constant  Value=[Jx+5e-2 Jy+5e-2 Jz+1e-1]
  Mbx : Product
  Mby : Product
  Mbz : Product
  Multiply : Product  Multiplication=Matrix(*)
  Multiply1 : Product  Multiplication=Matrix(*)
  Multiply{2..16} (15 alike) : Product
  Multiply17 : Product  Multiplication=Matrix(*)
  Mux{,1..3} (4 alike) : Mux  Inputs=3
  Subtract : Sum  Inputs=+-
  Subtract1 : Sum
  Subtract2 : Sum  Inputs=-+
  Sum : Sum  Inputs=++-
  Sum1 : Sum
  Sum2 : Sum
  Terminator : Terminator
  Transpose : Math  Operator=transpose  SaturateOnIntegerOverflow=on
  Transpose1 : Math  Operator=transpose  SaturateOnIntegerOverflow=on
  buoyangcy rho*g*V : Constant  Value=rho.water*g*V
  cos(phi) : Trigonometry  Operator=cos
  cos(theta) : Trigonometry  Operator=cos
  cos(theta)*cos(phi) : Product
  m*g : Constant  Value=[0 0 m*g]
  mg-rho*g*v : Constant  Value=rho.water*g*V
  sin(phi) : Trigonometry
  sin(theta) : Trigonometry
  xb : Constant  Value=buoPos.y
  xb*cos(theta)*cos(phi) : Product
  xb*cos(theta)*sin(phi) : Product  Inputs=3
  yb : Constant  Value=buoPos.y
  yb*cos(theta)*cos(phi) : Product
  zb : Constant  Value=buoPos.z
  zb*cos(theta)*cos(phi) : Product
  zb*sin(theta) : Product
  Fb : Outport
  Mb : Outport  Port=2
  wires:
  Demux/3 -> Mbz/1
  Demux1/2 -> Mby/2
  Demux/2 -> Mby/1
  Demux/1 -> Mbx/1
  Demux1/3 -> Mbz/2
  Demux1/1 -> Mbx/2
  aglAcc/1 -> Demux1/1
  J1/1 -> Demux/1
  Mby/1 -> Mux1/2
  Mbx/1 -> Mux1/1
  Mbz/1 -> Mux1/3
  Fe/1 -> Sum/2
  m*g/1 -> Sum/1
  Constant1/1 -> Fe/1
  posAcc/1 -> Fe/2
  Sum/1 -> Multiply/2
  Mux1/1 -> Multiply1/2
  mg-rho*g*v/1 -> Sum/3
  Bus Selector/2 -> Transpose/1  "<DCMbe>"
  Transpose/1 -> Multiply/1, Multiply1/1
  Multiply3/1 -> Multiply6/2
  Abs1/1 -> Multiply3/2
  Demux2/2 -> Multiply3/1, Abs1/1  "v"
  0.5*rho*Cd*Sz/1 -> Multiply7/1
  Abs/1 -> Multiply2/2
  Abs2/1 -> Multiply4/2
  Demux2/1 -> Multiply2/1, Abs/1  "u"
  Demux2/3 -> Abs2/1, Multiply4/1  "w"
  0.5*rho*Cd*Sy/1 -> Multiply6/1
  Multiply2/1 -> Multiply5/2
  Multiply4/1 -> Multiply7/2
  0.5*rho*Cd*Sx/1 -> Multiply5/1
  Multiply6/1 -> Mux/2
  Multiply5/1 -> Mux/1
  Multiply7/1 -> Mux/3
  Mux/1 -> F-Fd/1
  Multiply/1 -> F-Fd/2
  F-Fd/1 -> Fb/1
  Bus Selector/1 -> Demux2/1  "<Vb>"
  body states/1 -> [bodyStates], Bus Selector/1
  Dx/1 -> Multiply11/1
  Demux3/2 -> Abs4/1, Multiply9/1  "q"
  Bus Selector1/2 -> Demux3/1  "<Wb>"
  Demux3/1 -> Multiply8/1, Abs3/1  "p"
  Dy/1 -> Multiply12/1
  Multiply9/1 -> Multiply12/2
  Abs4/1 -> Multiply9/2
  Abs5/1 -> Multiply10/2
  Demux3/3 -> Abs5/1, Multiply10/1  "r"
  Abs3/1 -> Multiply8/2
  Multiply8/1 -> Multiply11/2
  Multiply10/1 -> Multiply13/2
  Dz/1 -> Multiply13/1
  [bodyStates] -> Bus Selector1/1
  Multiply13/1 -> Mux2/3
  Multiply12/1 -> Mux2/2
  Multiply11/1 -> Mux2/1
  sin(theta)/1 -> -yb*sin(theta)/2, zb*sin(theta)/2
  Subtract1/1 -> Multiply14/2
  xb/1 -> xb*cos(theta)*sin(phi)/1, xb*cos(theta)*cos(phi)/2
  Gain/1 -> -yb*sin(theta)/1
  buoyangcy rho*g*V/1 -> Multiply15/1, Multiply14/1, Multiply16/1
  Subtract2/1 -> Multiply15/2
  yb/1 -> Gain/1, yb*cos(theta)*cos(phi)/2
  Demux4/1 -> cos(phi)/1, sin(phi)/1
  Demux4/2 -> sin(theta)/1, cos(theta)/1
  cos(theta)*cos(phi)/1 -> zb*cos(theta)*cos(phi)/2, xb*cos(theta)*cos(phi)/1, yb*cos(theta)*cos(phi)/1
  zb*sin(theta)/1 -> Subtract1/2
  sin(phi)/1 -> xb*cos(theta)*sin(phi)/2
  zb/1 -> zb*sin(theta)/1, zb*cos(theta)*cos(phi)/1
  zb*cos(theta)*cos(phi)/1 -> Subtract/1
  yb*cos(theta)*cos(phi)/1 -> Subtract/2
  xb*cos(theta)*sin(phi)/1 -> Subtract2/1
  Subtract/1 -> Multiply16/2
  -yb*sin(theta)/1 -> Subtract2/2
  cos(phi)/1 -> cos(theta)*cos(phi)/1
  xb*cos(theta)*cos(phi)/1 -> Subtract1/1
  cos(theta)/1 -> xb*cos(theta)*sin(phi)/3, cos(theta)*cos(phi)/2
  Bus Selector1/3 -> Demux4/1  "<angle>"
  Demux4/3 -> Terminator/1
  Multiply14/1 -> Mux3/2
  Multiply16/1 -> Mux3/1
  Multiply15/1 -> Mux3/3
  Mux2/1 -> Sum1/1
  Mux3/1 -> Sum1/2
  Sum1/1 -> Gain1/1
  Bus Selector1/1 -> Transpose1/1  "<DCMbe>"
  Transpose1/1 -> Multiply17/1
  Gain1/1 -> Multiply17/2
  Multiply1/1 -> Sum2/1
  Multiply17/1 -> Sum2/2
  Sum2/1 -> Mb/1
